simulink model "fixed_time_MASs"  (R2023b)
settings: Solver=FixedStepAuto  StartTime=0.0  StopTime=20  FixedStep=0.0001  RelTol=1e-3
(part 2 of 2)

== matlab function fixed_time_MASs/Subsystem/MATLAB Function9 ==
  data: t input; y output
function y = fcn(t)
if t<5
    y = 1;
else
    y = 0.7+0.3*(exp(-(t-5)));
end

== matlab function fixed_time_MASs/Subsystem1/MATLAB Function11 ==
  data: d2 input; u input; y output; m input; r input
function y = fcn(d2, u, m, r)

y = d2-(1-m)*u+r;

== matlab function fixed_time_MASs/Subsystem1/MATLAB Function12 ==
  data: t input; y output; x1 input; x2 input
function y = fcn(t, x1, x2)
y=5*cos(t)+0.6*sin(x1)*cos(x2/3);

== matlab function fixed_time_MASs/Subsystem1/MATLAB Function13 ==
  data: u input; y output; m input; r input
function y = fcn(u, m, r)
y=m*u+r;

== matlab function fixed_time_MASs/Subsystem1/MATLAB Function3 ==
  data: d1_hat output; x1 input; x2 input; xi_1 output; xi_1k input
function [d1_hat, xi_1] = fcn(x1, x2, xi_1k)

f1 = 0.2*x1*sin(x1*x1);
fi0 = 1; fi1 = 5; fi2 = 5;
% a1 = 123; q1 = 101; 
% h1 = 91; n1 = 101;
a1 = 7; q1 = 10; 
h1 = 13; n1 = 10;
Ts = 0.0001;

xi_1 = xi_1k+Ts*(x2+f1-fi0*(xi_1k-x1)-fi1*(abs(xi_1k-x1)^(a1/q1))*sign(xi_1k-x1)-fi2*(abs(xi_1k-x1)^(h1/n1))*sign(xi_1k-x1));
d1_hat = -fi0*(xi_1k-x1)-fi1*(abs(xi_1k-x1)^(a1/q1))*sign(xi_1k-x1)-fi2*(abs(xi_1k-x1)^(h1/n1))*sign(xi_1k-x1);

== matlab function fixed_time_MASs/MATLAB Function1 ==
  data: t input; x1d output; a input; b input; dx1d output; ddx1d output
function [x1d, dx1d, ddx1d] = fcn(t,a,b)
x1d = sin(a*t)+1.5*sin(b*t);
dx1d = a*cos(a*t)+1.5*b*cos(b*t);
ddx1d = -a*a*sin(a*t)-b*b*1.5*sin(b*t);

== matlab function fixed_time_MASs/Subsystem1/MATLAB Function1 ==
  data: t input; x1d output; a input; b input; dx1d output; ddx1d output; data input
function [x1d, dx1d, ddx1d] = fcn(t,a,b, data)
% x1d = sin(a*t)+1.5*sin(b*t);
x1d = data;
dx1d = a*cos(a*t)+1.5*b*cos(b*t);
ddx1d = -a*a*sin(a*t)-b*b*1.5*sin(b*t);

== matlab function fixed_time_MASs/Subsystem/MATLAB Function14 ==
  settings: updateMethod=DISCRETE
  data: x2 input; xi_2k input; alph1 input; u output; alph2 input
function u = fcn(x2, xi_2k, alph1, alph2)
persistent u_last k
if isempty(u_last); u_last = 0; end
if isempty(k); k = 0; end

DETA = 4; theta = 0.1; tuta = 0.1; v1_bar = 0.07; v2_bar = 0.25; v1 = 0.01; v2 = 0.01;

e2 = x2+xi_2k-alph1;
if abs(u_last) <= DETA
    wt = -alph2*(tanh(e2*alph2/theta))*(1+tuta)-v1_bar*(tanh(e2*v1_bar/theta))*(1+tuta);
else
    wt = alph2-v2_bar*tanh(e2*v2_bar/theta);
end


psi = wt - u_last;
triggered = 0;
if abs(u_last) <= DETA
    if abs(psi) >= (v1 + tuta * abs(u_last))
        triggered = 1;
    end
else
    if abs(psi) >= v2
        triggered = 1;
    end
end

if triggered
    u_last = wt;
end

u = u_last;

== matlab function fixed_time_MASs/Subsystem3/MATLAB Function5 ==
  data: t input; x1d output; a input; b input; dx1d output; ddx1d output; data input
function [x1d, dx1d, ddx1d] = fcn(t,a,b, data)
% x1d = sin(a*t)+1.5*sin(b*t);
x1d = data;
dx1d = a*cos(a*t)+1.5*b*cos(b*t);
ddx1d = -a*a*sin(a*t)-b*b*1.5*sin(b*t);

== matlab function fixed_time_MASs/Subsystem3/MATLAB Function7 ==
  data: t input; x1d output; dx1d output; ddx1d output; a input; data input
function [x1d, dx1d, ddx1d] = fcn(t,a, data)
% if t<5
%     x1d = 0;
% else
%     x1d = a;
% end
x1d = data;
dx1d = 0;
ddx1d = 0;

== matlab function fixed_time_MASs/Subsystem3/MATLAB Function1 ==
  data: d1_hat output; x1 input; x2 input; xi_1 output; xi_1k input
function [d1_hat, xi_1] = fcn(x1, x2, xi_1k)

f1 = x1*sin(x1*x1);
fi0 = 1; fi1 = 5; fi2 = 5;
% a1 = 123; q1 = 101; 
% h1 = 91; n1 = 101;
a1 = 7; q1 = 10; 
h1 = 13; n1 = 10;
Ts = 0.0001;

xi_1 = xi_1k+Ts*(x2+f1-fi0*(xi_1k-x1)-fi1*(abs(xi_1k-x1)^(a1/q1))*sign(xi_1k-x1)-fi2*(abs(xi_1k-x1)^(h1/n1))*sign(xi_1k-x1));
d1_hat = -fi0*(xi_1k-x1)-fi1*(abs(xi_1k-x1)^(a1/q1))*sign(xi_1k-x1)-fi2*(abs(xi_1k-x1)^(h1/n1))*sign(xi_1k-x1);

== matlab function fixed_time_MASs/Subsystem1/MATLAB Function2 ==
  data: t input; x1d output; dx1d output; ddx1d output; a input; data input
function [x1d, dx1d, ddx1d] = fcn(t,a, data)
% if t<5
%     x1d = 0;
% else
%     x1d = a;
% end
x1d = data;
dx1d = 0;
ddx1d = 0;

== matlab function fixed_time_MASs/Subsystem2/MATLAB Function5 ==
  data: t input; x1d output; a input; b input; dx1d output; ddx1d output; data input
function [x1d, dx1d, ddx1d] = fcn(t,a,b, data)
% x1d = sin(a*t)+1.5*sin(b*t);
x1d = data;
dx1d = a*cos(a*t)+1.5*b*cos(b*t);
ddx1d = -a*a*sin(a*t)-b*b*1.5*sin(b*t);

== matlab function fixed_time_MASs/Subsystem2/MATLAB Function7 ==
  data: t input; x1d output; dx1d output; ddx1d output; a input; data input
function [x1d, dx1d, ddx1d] = fcn(t,a, data)
% if t<5
%     x1d = 0;
% else
%     x1d = a;
% end
x1d = data;
dx1d = 0;
ddx1d = 0;

== matlab function fixed_time_MASs/Subsystem2/MATLAB Function1 ==
  data: d1_hat output; x1 input; x2 input; xi_1 output; xi_1k input
function [d1_hat, xi_1] = fcn(x1, x2, xi_1k)

f1 = 0.5*x1*sin(x1*x1);
fi0 = 1; fi1 = 5; fi2 = 5;
% a1 = 123; q1 = 101; 
% h1 = 91; n1 = 101;
a1 = 7; q1 = 10; 
h1 = 13; n1 = 10;
Ts = 0.0001;

xi_1 = xi_1k+Ts*(x2+f1-fi0*(xi_1k-x1)-fi1*(abs(xi_1k-x1)^(a1/q1))*sign(xi_1k-x1)-fi2*(abs(xi_1k-x1)^(h1/n1))*sign(xi_1k-x1));
d1_hat = -fi0*(xi_1k-x1)-fi1*(abs(xi_1k-x1)^(a1/q1))*sign(xi_1k-x1)-fi2*(abs(xi_1k-x1)^(h1/n1))*sign(xi_1k-x1);

== matlab function fixed_time_MASs/Subsystem1/MATLAB Function9 ==
  data: t input; y output
function y = fcn(t)
if t<5
    y = 1;
else
    y = 0.7+0.3*(exp(-(t-5)));
end

== matlab function fixed_time_MASs/MATLAB Function ==
  data: x1d input; u0 output; dx1d input; ddx1d input; x1 input; x2 input
function u0 = fcn(x1d, dx1d, ddx1d, x1, x2)
A1 = 100; A2 = 190;
f1 = x1*sin(x1*x1);
f2 = x1*x2*x2;
g1 = 1; g2 = 1;
z1 = x1d - x1;
v1 = (dx1d-f1+A1*z1)/g1;
z2 = v1 - x2;
dz1 = -A1*z1+g1*z2;
df1 = sin(x1*x1)+2*x1*x1*cos(x1*x1);
dv1 = ddx1d/g1-df1/g1+A1*dz1/g1;
u0 = (z1*g1+dv1-f2+A2*z2)/g2;

== matlab function fixed_time_MASs/Subsystem2/MATLAB Function14 ==
  settings: updateMethod=DISCRETE
  data: x2 input; xi_2k input; alph1 input; u output; alph2 input
function u = fcn(x2, xi_2k, alph1, alph2)
persistent u_last k
if isempty(u_last); u_last = 0; end
if isempty(k); k = 0; end

DETA = 4; theta = 0.1; tuta = 0.1; v1_bar = 0.07; v2_bar = 0.25; v1 = 0.01; v2 = 0.01;

e2 = x2+xi_2k-alph1;
if abs(u_last) <= DETA
    wt = -alph2*(tanh(e2*alph2/theta))*(1+tuta)-v1_bar*(tanh(e2*v1_bar/theta))*(1+tuta);
else
    wt = alph2-v2_bar*tanh(e2*v2_bar/theta);
end


psi = wt - u_last;
triggered = 0;
if abs(u_last) <= DETA
    if abs(psi) >= (v1 + tuta * abs(u_last))
        triggered = 1;
    end
else
    if abs(psi) >= v2
        triggered = 1;
    end
end

if triggered
    u_last = wt;
end

u = u_last;

== matlab function fixed_time_MASs/Subsystem2/MATLAB Function10 ==
  data: u input; y output
function y = fcn(u)

y = sin(0.7*u)*(exp(0.5*cos(0.7*u)));

== matlab function fixed_time_MASs/Subsystem2/MATLAB Function11 ==
  data: d2 input; u input; y output; m input; r input
function y = fcn(d2, u, m, r)

y = d2-(1-m)*u+r;

== matlab function fixed_time_MASs/Subsystem2/MATLAB Function12 ==
  data: t input; y output; x1 input; x2 input
function y = fcn(t, x1, x2)
y=5*cos(t)+0.6*sin(x1)*cos(x2/3);

== matlab function fixed_time_MASs/Subsystem2/MATLAB Function13 ==
  data: u input; y output; m input; r input
function y = fcn(u, m, r)
y=m*u+r;

== matlab function fixed_time_MASs/Subsystem3/MATLAB Function14 ==
  settings: updateMethod=DISCRETE
  data: x2 input; xi_2k input; alph1 input; u output; alph2 input
function u = fcn(x2, xi_2k, alph1, alph2)
persistent u_last k
if isempty(u_last); u_last = 0; end
if isempty(k); k = 0; end

DETA = 4; theta = 0.1; tuta = 0.1; v1_bar = 0.07; v2_bar = 0.25; v1 = 0.01; v2 = 0.01;

e2 = x2+xi_2k-alph1;
if abs(u_last) <= DETA
    wt = -alph2*(tanh(e2*alph2/theta))*(1+tuta)-v1_bar*(tanh(e2*v1_bar/theta))*(1+tuta);
else
    wt = alph2-v2_bar*tanh(e2*v2_bar/theta);
end


psi = wt - u_last;
triggered = 0;
if abs(u_last) <= DETA
    if abs(psi) >= (v1 + tuta * abs(u_last))
        triggered = 1;
    end
else
    if abs(psi) >= v2
        triggered = 1;
    end
end

if triggered
    u_last = wt;
end

u = u_last;

== matlab function fixed_time_MASs/Subsystem4/MATLAB Function5 ==
  data: t input; x1d output; a input; b input; dx1d output; ddx1d output; data input
function [x1d, dx1d, ddx1d] = fcn(t,a,b, data)
% x1d = sin(a*t)+1.5*sin(b*t);
x1d = data;
dx1d = a*cos(a*t)+1.5*b*cos(b*t);
ddx1d = -a*a*sin(a*t)-b*b*1.5*sin(b*t);

== matlab function fixed_time_MASs/Subsystem4/MATLAB Function7 ==
  data: t input; x1d output; dx1d output; ddx1d output; a input; data input
function [x1d, dx1d, ddx1d] = fcn(t,a, data)
% if t<5
%     x1d = 0;
% else
%     x1d = a;
% end
x1d = data;
dx1d = 0;
ddx1d = 0;

== matlab function fixed_time_MASs/Subsystem4/MATLAB Function1 ==
  data: d1_hat output; x1 input; x2 input; xi_1 output; xi_1k input
function [d1_hat, xi_1] = fcn(x1, x2, xi_1k)

f1 = 1.2*x1*sin(x1*x1);
fi0 = 1; fi1 = 5; fi2 = 5;
% a1 = 123; q1 = 101; 
% h1 = 91; n1 = 101;
a1 = 7; q1 = 10; 
h1 = 13; n1 = 10;
Ts = 0.0001;

xi_1 = xi_1k+Ts*(x2+f1-fi0*(xi_1k-x1)-fi1*(abs(xi_1k-x1)^(a1/q1))*sign(xi_1k-x1)-fi2*(abs(xi_1k-x1)^(h1/n1))*sign(xi_1k-x1));
d1_hat = -fi0*(xi_1k-x1)-fi1*(abs(xi_1k-x1)^(a1/q1))*sign(xi_1k-x1)-fi2*(abs(xi_1k-x1)^(h1/n1))*sign(xi_1k-x1);

== matlab function fixed_time_MASs/Subsystem4/MATLAB Function14 ==
  settings: updateMethod=DISCRETE
  data: x2 input; xi_2k input; alph1 input; u output; alph2 input
function u = fcn(x2, xi_2k, alph1, alph2)
persistent u_last k
if isempty(u_last); u_last = 0; end
if isempty(k); k = 0; end

DETA = 4; theta = 0.1; tuta = 0.1; v1_bar = 0.07; v2_bar = 0.25; v1 = 0.01; v2 = 0.01;

e2 = x2+xi_2k-alph1;
if abs(u_last) <= DETA
    wt = -alph2*(tanh(e2*alph2/theta))*(1+tuta)-v1_bar*(tanh(e2*v1_bar/theta))*(1+tuta);
else
    wt = alph2-v2_bar*tanh(e2*v2_bar/theta);
end


psi = wt - u_last;
triggered = 0;
if abs(u_last) <= DETA
    if abs(psi) >= (v1 + tuta * abs(u_last))
        triggered = 1;
    end
else
    if abs(psi) >= v2
        triggered = 1;
    end
end

if triggered
    u_last = wt;
end

u = u_last;

== matlab function fixed_time_MASs/Subsystem1/MATLAB Function4 ==
  data: d2_hat output; x1 input; x2 input; u input; xi_2 output; xi_2k input
function [d2_hat, xi_2] = fcn(x1, x2, u, xi_2k)

f2 = 0.2*x1*x2*x2;
fi0 = 100; fi1 = 1; fi2 = 1;
% a1 = 123; q1 = 101; 
% h1 = 91; n1 = 101;
a1 = 7; q1 = 10; 
h1 = 13; n1 = 10;
Ts = 0.0001;

xi_2 = xi_2k+Ts*(u+f2-fi0*(xi_2k-x2)-fi1*(abs(xi_2k-x2)^(a1/q1))*sign(xi_2k-x2)-fi2*(abs(xi_2k-x2)^(h1/n1))*sign(xi_2k-x2));
d2_hat = -fi0*(xi_2k-x2)-fi1*(abs(xi_2k-x2)^(a1/q1))*sign(xi_2k-x2)-fi2*(abs(xi_2k-x2)^(h1/n1))*sign(xi_2k-x2);

== matlab function fixed_time_MASs/MATLAB Function2 ==
  data: t input; x1d output; dx1d output; ddx1d output; a input
function [x1d, dx1d, ddx1d] = fcn(t,a)
% if t<5
%     x1d = 0;
% elseif t>=5 && t<15
%     x1d = a;
% else
%     x1d = 0;
% end
if t<5
    x1d = 0;
else
    x1d = a;
end
dx1d = 0;
ddx1d = 0;

== matlab function fixed_time_MASs/Subsystem2/MATLAB Function9 ==
  data: t input; y output
function y = fcn(t)
if t<5
    y = 1;
else
    y = 0.7+0.3*(exp(-(t-5)));
end

== matlab function fixed_time_MASs/Subsystem1/MATLAB Function7 ==
  data: x1 input; xi_1 input; d1_hat input; xd input; alph1 output; dxd input
function alph1 = fcn(x1, xi_1, d1_hat, xd, dxd)
k1 = 50; c1 = 5; m1 = 0;
f1 = 0.2*x1*sin(x1*x1);
% a2 = 123; q2 = 101; 
% h2 = 91; n2 = 101;
a2 = 9; q2 = 10; 
h2 = 11; n2 = 10;

e1 = x1 - xd;
alph1 = -f1-m1*e1-k1*(abs(e1)^(a2/q2))*sign(e1)-c1*(abs(e1)^(h2/n2))*sign(e1)+dxd+xi_1-d1_hat;

== matlab function fixed_time_MASs/Subsystem3/MATLAB Function10 ==
  data: u input; y output
function y = fcn(u)

y = sin(0.7*u)*(exp(1*cos(0.7*u)));

== matlab function fixed_time_MASs/Subsystem3/MATLAB Function11 ==
  data: d2 input; u input; y output; m input; r input
function y = fcn(d2, u, m, r)

y = d2-(1-m)*u+r;

== matlab function fixed_time_MASs/Subsystem3/MATLAB Function12 ==
  data: t input; y output; x1 input; x2 input
function y = fcn(t, x1, x2)
y=5*cos(t)+0.6*sin(x1)*cos(x2/3);

== matlab function fixed_time_MASs/Subsystem3/MATLAB Function13 ==
  data: u input; y output; m input; r input
function y = fcn(u, m, r)
y=m*u+r;

== matlab function fixed_time_MASs/Subsystem1/MATLAB Function8 ==
  data: alph2 output; x1 input; x2 input; xd input; xi_2k input; d2_hat input; alph1 input; dalph1 input
function alph2 = fcn(x1, x2, xd, xi_2k, d2_hat, alph1, dalph1)
k2 = 55; c2 = 25; m2 = 0.5;

f2 = 0.2*x1*x2*x2;
% a2 = 123; q2 = 101; 
% h2 = 91; n2 = 101;
a2 = 9; q2 = 10; 
h2 = 11; n2 = 10;
elp = 0.1;

e1 = x1-xd;
e2 = x2+xi_2k-alph1;

alph2_bar = k2*(abs(e2)^(a2/q2))+c2*(abs(e2)^(h2/n2))+m2*e2+d2_hat+e1+f2-dalph1;
alph2 = -e2*alph2_bar*alph2_bar/((sqrt(e2*e2*alph2_bar*alph2_bar+elp*elp)));

== matlab function fixed_time_MASs/Subsystem2/MATLAB Function2 ==
  data: d2_hat output; x1 input; x2 input; u input; xi_2 output; xi_2k input
function [d2_hat, xi_2] = fcn(x1, x2, u, xi_2k)

f2 = 0.5*x1*x2*x2;
fi0 = 100; fi1 = 1; fi2 = 1;
% a1 = 123; q1 = 101; 
% h1 = 91; n1 = 101;
a1 = 7; q1 = 10; 
h1 = 13; n1 = 10;
Ts = 0.0001;

xi_2 = xi_2k+Ts*(u+f2-fi0*(xi_2k-x2)-fi1*(abs(xi_2k-x2)^(a1/q1))*sign(xi_2k-x2)-fi2*(abs(xi_2k-x2)^(h1/n1))*sign(xi_2k-x2));
d2_hat = -fi0*(xi_2k-x2)-fi1*(abs(xi_2k-x2)^(a1/q1))*sign(xi_2k-x2)-fi2*(abs(xi_2k-x2)^(h1/n1))*sign(xi_2k-x2);

== matlab function fixed_time_MASs/Subsystem2/MATLAB Function3 ==
  data: x1 input; xi_1 input; d1_hat input; xd input; alph1 output; dxd input
function alph1 = fcn(x1, xi_1, d1_hat, xd, dxd)
k1 = 50; c1 = 5; m1 = 0;
f1 = 0.5*x1*sin(x1*x1);
% a2 = 123; q2 = 101; 
% h2 = 91; n2 = 101;
a2 = 9; q2 = 10; 
h2 = 11; n2 = 10;

e1 = x1 - xd;
alph1 = -f1-m1*e1-k1*(abs(e1)^(a2/q2))*sign(e1)-c1*(abs(e1)^(h2/n2))*sign(e1)+dxd+xi_1-d1_hat;

== matlab function fixed_time_MASs/Subsystem2/MATLAB Function8 ==
  data: alph2 output; x1 input; x2 input; xd input; xi_2k input; d2_hat input; alph1 input; dalph1 input
function alph2 = fcn(x1, x2, xd, xi_2k, d2_hat, alph1, dalph1)
k2 = 55; c2 = 25; m2 = 0.5;

f2 = 0.5*x1*x2*x2;
% a2 = 123; q2 = 101; 
% h2 = 91; n2 = 101;
a2 = 9; q2 = 10; 
h2 = 11; n2 = 10;
elp = 0.1;

e1 = x1-xd;
e2 = x2+xi_2k-alph1;

alph2_bar = k2*(abs(e2)^(a2/q2))+c2*(abs(e2)^(h2/n2))+m2*e2+d2_hat+e1+f2-dalph1;
alph2 = -e2*alph2_bar*alph2_bar/((sqrt(e2*e2*alph2_bar*alph2_bar+elp*elp)));

== matlab function fixed_time_MASs/Subsystem/MATLAB Function5 ==
  data: t input; x1d output; a input; b input; dx1d output; ddx1d output; data input
function [x1d, dx1d, ddx1d] = fcn(t,a,b, data)
% x1d = sin(a*t)+1.5*sin(b*t);
x1d = data;
dx1d = a*cos(a*t)+1.5*b*cos(b*t);
ddx1d = -a*a*sin(a*t)-b*b*1.5*sin(b*t);

== matlab function fixed_time_MASs/Subsystem/MATLAB Function2 ==
  data: d2_hat output; x1 input; x2 input; u input; xi_2 output; xi_2k input
function [d2_hat, xi_2] = fcn(x1, x2, u, xi_2k)

f2 = 0.8*x1*x2*x2;
fi0 = 100; fi1 = 1; fi2 = 1;
% a1 = 123; q1 = 101; 
% h1 = 91; n1 = 101;
a1 = 7; q1 = 10; 
h1 = 13; n1 = 10;
Ts = 0.0001;

xi_2 = xi_2k+Ts*(u+f2-fi0*(xi_2k-x2)-fi1*(abs(xi_2k-x2)^(a1/q1))*sign(xi_2k-x2)-fi2*(abs(xi_2k-x2)^(h1/n1))*sign(xi_2k-x2));
d2_hat = -fi0*(xi_2k-x2)-fi1*(abs(xi_2k-x2)^(a1/q1))*sign(xi_2k-x2)-fi2*(abs(xi_2k-x2)^(h1/n1))*sign(xi_2k-x2);

== matlab function fixed_time_MASs/Subsystem/MATLAB Function3 ==
  data: x1 input; xi_1 input; d1_hat input; xd input; alph1 output; dxd input
function alph1 = fcn(x1, xi_1, d1_hat, xd, dxd)
k1 = 50; c1 = 5; m1 = 0;
f1 = 0.8*x1*sin(x1*x1);
% a2 = 123; q2 = 101; 
% h2 = 91; n2 = 101;
a2 = 9; q2 = 10; 
h2 = 11; n2 = 10;

e1 = x1 - xd;
alph1 = -f1-m1*e1-k1*(abs(e1)^(a2/q2))*sign(e1)-c1*(abs(e1)^(h2/n2))*sign(e1)+dxd+xi_1-d1_hat;

== matlab function fixed_time_MASs/Subsystem3/MATLAB Function9 ==
  data: t input; y output
function y = fcn(t)
if t<5
    y = 1;
else
    y = 0.7+0.3*(exp(-(t-5)));
end

== matlab function fixed_time_MASs/Subsystem/MATLAB Function8 ==
  data: alph2 output; x1 input; x2 input; xd input; xi_2k input; d2_hat input; alph1 input; dalph1 input
function alph2 = fcn(x1, x2, xd, xi_2k, d2_hat, alph1, dalph1)
k2 = 55; c2 = 25; m2 = 0.5;

f2 = 0.8*x1*x2*x2;
% a2 = 123; q2 = 101; 
% h2 = 91; n2 = 101;
a2 = 9; q2 = 10; 
h2 = 11; n2 = 10;
elp = 0.1;

e1 = x1-xd;
e2 = x2+xi_2k-alph1;

alph2_bar = k2*(abs(e2)^(a2/q2))+c2*(abs(e2)^(h2/n2))+m2*e2+d2_hat+e1+f2-dalph1;
alph2 = -e2*alph2_bar*alph2_bar/((sqrt(e2*e2*alph2_bar*alph2_bar+elp*elp)));

== matlab function fixed_time_MASs/Subsystem4/MATLAB Function10 ==
  data: u input; y output
function y = fcn(u)

y = sin(0.7*u)*(exp(1.2*cos(0.7*u)));

== matlab function fixed_time_MASs/Subsystem4/MATLAB Function11 ==
  data: d2 input; u input; y output; m input; r input
function y = fcn(d2, u, m, r)

y = d2-(1-m)*u+r;

== matlab function fixed_time_MASs/Subsystem4/MATLAB Function12 ==
  data: t input; y output; x1 input; x2 input
function y = fcn(t, x1, x2)
y=5*cos(t)+0.6*sin(x1)*cos(x2/3);

== matlab function fixed_time_MASs/Subsystem4/MATLAB Function13 ==
  data: u input; y output; m input; r input
function y = fcn(u, m, r)
y=m*u+r;

== matlab function fixed_time_MASs/Subsystem3/MATLAB Function2 ==
  data: d2_hat output; x1 input; x2 input; u input; xi_2 output; xi_2k input
function [d2_hat, xi_2] = fcn(x1, x2, u, xi_2k)

f2 = x1*x2*x2;
fi0 = 100; fi1 = 1; fi2 = 1;
% a1 = 123; q1 = 101; 
% h1 = 91; n1 = 101;
a1 = 7; q1 = 10; 
h1 = 13; n1 = 10;
Ts = 0.0001;

xi_2 = xi_2k+Ts*(u+f2-fi0*(xi_2k-x2)-fi1*(abs(xi_2k-x2)^(a1/q1))*sign(xi_2k-x2)-fi2*(abs(xi_2k-x2)^(h1/n1))*sign(xi_2k-x2));
d2_hat = -fi0*(xi_2k-x2)-fi1*(abs(xi_2k-x2)^(a1/q1))*sign(xi_2k-x2)-fi2*(abs(xi_2k-x2)^(h1/n1))*sign(xi_2k-x2);

== matlab function fixed_time_MASs/Subsystem3/MATLAB Function3 ==
  data: x1 input; xi_1 input; d1_hat input; xd input; alph1 output; dxd input
function alph1 = fcn(x1, xi_1, d1_hat, xd, dxd)
k1 = 50; c1 = 5; m1 = 0;
f1 = x1*sin(x1*x1);
% a2 = 123; q2 = 101; 
% h2 = 91; n2 = 101;
a2 = 9; q2 = 10; 
h2 = 11; n2 = 10;

e1 = x1 - xd;
alph1 = -f1-m1*e1-k1*(abs(e1)^(a2/q2))*sign(e1)-c1*(abs(e1)^(h2/n2))*sign(e1)+dxd+xi_1-d1_hat;

== matlab function fixed_time_MASs/Subsystem3/MATLAB Function8 ==
  data: alph2 output; x1 input; x2 input; xd input; xi_2k input; d2_hat input; alph1 input; dalph1 input
function alph2 = fcn(x1, x2, xd, xi_2k, d2_hat, alph1, dalph1)
k2 = 55; c2 = 25; m2 = 0.5;

f2 = x1*x2*x2;
% a2 = 123; q2 = 101; 
% h2 = 91; n2 = 101;
a2 = 9; q2 = 10; 
h2 = 11; n2 = 10;
elp = 0.1;

e1 = x1-xd;
e2 = x2+xi_2k-alph1;

alph2_bar = k2*(abs(e2)^(a2/q2))+c2*(abs(e2)^(h2/n2))+m2*e2+d2_hat+e1+f2-dalph1;
alph2 = -e2*alph2_bar*alph2_bar/((sqrt(e2*e2*alph2_bar*alph2_bar+elp*elp)));

== matlab function fixed_time_MASs/Subsystem4/MATLAB Function2 ==
  data: d2_hat output; x1 input; x2 input; u input; xi_2 output; xi_2k input
function [d2_hat, xi_2] = fcn(x1, x2, u, xi_2k)

f2 = 1.2*x1*x2*x2;
fi0 = 100; fi1 = 1; fi2 = 1;
% a1 = 123; q1 = 101; 
% h1 = 91; n1 = 101;
a1 = 7; q1 = 10; 
h1 = 13; n1 = 10;
Ts = 0.0001;

xi_2 = xi_2k+Ts*(u+f2-fi0*(xi_2k-x2)-fi1*(abs(xi_2k-x2)^(a1/q1))*sign(xi_2k-x2)-fi2*(abs(xi_2k-x2)^(h1/n1))*sign(xi_2k-x2));
d2_hat = -fi0*(xi_2k-x2)-fi1*(abs(xi_2k-x2)^(a1/q1))*sign(xi_2k-x2)-fi2*(abs(xi_2k-x2)^(h1/n1))*sign(xi_2k-x2);

== matlab function fixed_time_MASs/Subsystem1/MATLAB Function14 ==
  settings: updateMethod=DISCRETE
  data: x2 input; xi_2k input; alph1 input; u output; alph2 input
function u = fcn(x2, xi_2k, alph1, alph2)
persistent u_last k
if isempty(u_last); u_last = 0; end
if isempty(k); k = 0; end

DETA = 4; theta = 0.1; tuta = 0.1; v1_bar = 0.07; v2_bar = 0.25; v1 = 0.01; v2 = 0.01;

e2 = x2+xi_2k-alph1;
if abs(u_last) <= DETA
    wt = -alph2*(tanh(e2*alph2/theta))*(1+tuta)-v1_bar*(tanh(e2*v1_bar/theta))*(1+tuta);
else
    wt = alph2-v2_bar*tanh(e2*v2_bar/theta);
end


psi = wt - u_last;
triggered = 0;
if abs(u_last) <= DETA
    if abs(psi) >= (v1 + tuta * abs(u_last))
        triggered = 1;
    end
else
    if abs(psi) >= v2
        triggered = 1;
    end
end

if triggered
    u_last = wt;
end

u = u_last;

== matlab function fixed_time_MASs/Subsystem4/MATLAB Function3 ==
  data: x1 input; xi_1 input; d1_hat input; xd input; alph1 output; dxd input
function alph1 = fcn(x1, xi_1, d1_hat, xd, dxd)
k1 = 50; c1 = 5; m1 = 0;
f1 = 1.2*x1*sin(x1*x1);
% a2 = 123; q2 = 101; 
% h2 = 91; n2 = 101;
a2 = 9; q2 = 10; 
h2 = 11; n2 = 10;

e1 = x1 - xd;
alph1 = -f1-m1*e1-k1*(abs(e1)^(a2/q2))*sign(e1)-c1*(abs(e1)^(h2/n2))*sign(e1)+dxd+xi_1-d1_hat;

== matlab function fixed_time_MASs/Subsystem4/MATLAB Function8 ==
  data: alph2 output; x1 input; x2 input; xd input; xi_2k input; d2_hat input; alph1 input; dalph1 input
function alph2 = fcn(x1, x2, xd, xi_2k, d2_hat, alph1, dalph1)
k2 = 55; c2 = 25; m2 = 0.5;

f2 = 1.2*x1*x2*x2;
% a2 = 123; q2 = 101; 
% h2 = 91; n2 = 101;
a2 = 9; q2 = 10; 
h2 = 11; n2 = 10;
elp = 0.1;

e1 = x1-xd;
e2 = x2+xi_2k-alph1;

alph2_bar = k2*(abs(e2)^(a2/q2))+c2*(abs(e2)^(h2/n2))+m2*e2+d2_hat+e1+f2-dalph1;
alph2 = -e2*alph2_bar*alph2_bar/((sqrt(e2*e2*alph2_bar*alph2_bar+elp*elp)));

== matlab function fixed_time_MASs/Subsystem4/MATLAB Function9 ==
  data: t input; y output
function y = fcn(t)
if t<5
    y = 1;
else
    y = 0.7+0.3*(exp(-(t-5)));
end

== matlab function fixed_time_MASs/Subsystem/MATLAB Function10 ==
  data: u input; y output
function y = fcn(u)

y = sin(0.7*u)*(exp(0.8*cos(0.7*u)));

== matlab function fixed_time_MASs/Subsystem1/MATLAB Function10 ==
  data: u input; y output
function y = fcn(u)

y = sin(0.7*u)*(exp(0.2*cos(0.7*u)));

== matlab function fixed_time_MASs/Subsystem/MATLAB Function11 ==
  data: d2 input; u input; y output; m input; r input
function y = fcn(d2, u, m, r)

y = d2-(1-m)*u+r;

== matlab function fixed_time_MASs/Subsystem/MATLAB Function12 ==
  data: t input; y output; x1 input; x2 input
function y = fcn(t, x1, x2)
y=5*cos(t)+0.6*sin(x1)*cos(x2/3);
